simulink model "VCU_CS75_12_27_test"  (R2014a)
settings: Solver=FixedStepDiscrete  StartTime=0.0  StopTime=25  FixedStep=0.0005  RelTol=1e-3
undefined symbols (not defined in the file): D1, D2, D3, ecucoder_acal, ErrorSumMax1, ErrorSumMax2, ErrorSumMax3, I1, I2, I3, I_SW01_L, LaterlAngleCommand, LDW, P1, P2, P3, RemoteAcclPosition
libraries: simulink x913, ec5744lib x39
(part 3 of 30)

== system VCU_CS75_12_27_test/长安CS75底盘程序，20ms一次/Output/Subsystem/TransmitMessages11 ==
  GW_LCDAL_2EA : Subsystem
  GW_LCDAL_2EA_Ter : Terminator
  LCDAL_AudioWarningEnableStatus : Ground
  LCDAL_BSDLCAAlert : Ground
  LCDAL_BSDLCAEnableStatus : Ground
  LCDAL_BSDLCAStatus : Ground
  LCDAL_CTAAlert : Ground
  LCDAL_CTAEnableStatus : Ground
  LCDAL_CTAStatus : Ground
  LCDAL_LCATTCSettingStatus : Ground
  LCDAL_LockCtrlEnableStatus : Ground
  LCDAL_RCWAlert : Ground
  LCDAL_RCWEnableStatus : Ground
  LCDAL_RCWSoundEnableStatus : Ground
  LCDAL_RCWStatus : Ground
  LCDAL_SEAAlert : Ground
  LCDAL_SEAEnableStatus : Ground
  LCDAL_SEAStatus : Ground
  LCDAL_SystemStatus : Ground
  wires:
  GW_LCDAL_2EA/1(output) -> GW_LCDAL_2EA_Ter/1
  LCDAL_LCATTCSettingStatus/1 -> GW_LCDAL_2EA/17(LCDAL_LCATTCSettingStatus_in)
  LCDAL_LockCtrlEnableStatus/1 -> GW_LCDAL_2EA/16(LCDAL_LockCtrlEnableStatus_in)
  LCDAL_AudioWarningEnableStatus/1 -> GW_LCDAL_2EA/15(LCDAL_AudioWarningEnableStatus_in)
  LCDAL_SEAStatus/1 -> GW_LCDAL_2EA/14(LCDAL_SEAStatus_in)
  LCDAL_SEAAlert/1 -> GW_LCDAL_2EA/13(LCDAL_SEAAlert_in)
  LCDAL_SEAEnableStatus/1 -> GW_LCDAL_2EA/12(LCDAL_SEAEnableStatus_in)
  LCDAL_RCWSoundEnableStatus/1 -> GW_LCDAL_2EA/11(LCDAL_RCWSoundEnableStatus_in)
  LCDAL_RCWStatus/1 -> GW_LCDAL_2EA/10(LCDAL_RCWStatus_in)
  LCDAL_RCWAlert/1 -> GW_LCDAL_2EA/9(LCDAL_RCWAlert_in)
  LCDAL_RCWEnableStatus/1 -> GW_LCDAL_2EA/8(LCDAL_RCWEnableStatus_in)
  LCDAL_CTAStatus/1 -> GW_LCDAL_2EA/7(LCDAL_CTAStatus_in)
  LCDAL_CTAAlert/1 -> GW_LCDAL_2EA/6(LCDAL_CTAAlert_in)
  LCDAL_CTAEnableStatus/1 -> GW_LCDAL_2EA/5(LCDAL_CTAEnableStatus_in)
  LCDAL_BSDLCAStatus/1 -> GW_LCDAL_2EA/4(LCDAL_BSDLCAStatus_in)
  LCDAL_BSDLCAAlert/1 -> GW_LCDAL_2EA/3(LCDAL_BSDLCAAlert_in)
  LCDAL_BSDLCAEnableStatus/1 -> GW_LCDAL_2EA/2(LCDAL_BSDLCAEnableStatus_in)
  LCDAL_SystemStatus/1 -> GW_LCDAL_2EA/1(LCDAL_SystemStatus_in)

== system VCU_CS75_12_27_test/长安CS75底盘程序，20ms一次/Output/Subsystem/TransmitMessages13 ==
  GW_LCDAR_2FA : Subsystem
  GW_LCDAR_2FA_Ter : Terminator
  LCDAR_BSDLCAAlert : Ground
  LCDAR_BSDLCAStatus : Ground
  LCDAR_CTAAlert : Ground
  LCDAR_CTAStatus : Ground
  LCDAR_RCWAlert : Ground
  LCDAR_RCWStatus : Ground
  LCDAR_SEAAlert : Ground
  LCDAR_SEAStatus : Ground
  LCDAR_SystemStatus : Ground
  wires:
  LCDAR_SystemStatus/1 -> GW_LCDAR_2FA/1(LCDAR_SystemStatus_in)
  LCDAR_BSDLCAAlert/1 -> GW_LCDAR_2FA/2(LCDAR_BSDLCAAlert_in)
  LCDAR_BSDLCAStatus/1 -> GW_LCDAR_2FA/3(LCDAR_BSDLCAStatus_in)
  LCDAR_CTAAlert/1 -> GW_LCDAR_2FA/4(LCDAR_CTAAlert_in)
  LCDAR_CTAStatus/1 -> GW_LCDAR_2FA/5(LCDAR_CTAStatus_in)
  LCDAR_RCWAlert/1 -> GW_LCDAR_2FA/6(LCDAR_RCWAlert_in)
  LCDAR_RCWStatus/1 -> GW_LCDAR_2FA/7(LCDAR_RCWStatus_in)
  LCDAR_SEAAlert/1 -> GW_LCDAR_2FA/8(LCDAR_SEAAlert_in)
  LCDAR_SEAStatus/1 -> GW_LCDAR_2FA/9(LCDAR_SEAStatus_in)
  GW_LCDAR_2FA/1(output) -> GW_LCDAR_2FA_Ter/1

== system VCU_CS75_12_27_test/长安CS75底盘程序，20ms一次/Output/Subsystem/TransmitMessages14 ==
  CRC : Ground
  LAS_2AD : Subsystem
  LAS_2AD_Ter : Terminator
  LAS_DriverHandsOff : Ground
  LAS_IACCMode : Ground
  LAS_IACCTextInfoForDriver : Ground
  LAS_TargetBasedLateralCOntrol : Ground
  RollingConter : Ground
  wires:
  LAS_2AD/1(output) -> LAS_2AD_Ter/1
  CRC/1 -> LAS_2AD/6(CRC_in)
  RollingConter/1 -> LAS_2AD/5(RollingConter_in)
  LAS_IACCTextInfoForDriver/1 -> LAS_2AD/4(LAS_IACCTextInfoForDriver_in)
  LAS_IACCMode/1 -> LAS_2AD/3(LAS_IACCMode_in)
  LAS_DriverHandsOff/1 -> LAS_2AD/2(LAS_DriverHandsOff_in)
  LAS_TargetBasedLateralCOntrol/1 -> LAS_2AD/1(LAS_TargetBasedLateralCOntrol_in)

== system VCU_CS75_12_27_test/长安CS75底盘程序，20ms一次/Output/Subsystem/TransmitMessages2 ==
  ACC_3C5 : Subsystem
  ACC_3C5_Ter : Terminator
  ACC_TargetRange : Ground
  ACC_TargetType : Ground
  CRC : Ground
  RollingConter : Ground
  wires:
  ACC_TargetRange/1 -> ACC_3C5/1(ACC_TargetRange_in)
  ACC_TargetType/1 -> ACC_3C5/2(ACC_TargetType_in)
  RollingConter/1 -> ACC_3C5/3(RollingConter_in)
  CRC/1 -> ACC_3C5/4(CRC_in)
  ACC_3C5/1(output) -> ACC_3C5_Ter/1

== system VCU_CS75_12_27_test/长安CS75底盘程序，20ms一次/Output/Subsystem/TransmitMessages3 ==
  ACC_3D5 : Subsystem
  ACC_3D5_Ter : Terminator
  ACC_LeftTargetDection : Ground
  ACC_LeftTargetLatRange : Ground
  ACC_LeftTargetLngRange : Ground
  ACC_LeftTargetType : Ground
  ACC_RightTargetDection : Ground
  ACC_RightTargetLatRange : Ground
  ACC_RightTargetLngRange : Ground
  ACC_RightTargetType : Ground
  CRC : Ground
  RollingConter : Ground
  wires:
  ACC_LeftTargetLngRange/1 -> ACC_3D5/1(ACC_LeftTargetLngRange_in)
  ACC_RightTargetDection/1 -> ACC_3D5/2(ACC_RightTargetDection_in)
  ACC_LeftTargetDection/1 -> ACC_3D5/3(ACC_LeftTargetDection_in)
  ACC_LeftTargetType/1 -> ACC_3D5/4(ACC_LeftTargetType_in)
  ACC_LeftTargetLatRange/1 -> ACC_3D5/5(ACC_LeftTargetLatRange_in)
  ACC_RightTargetType/1 -> ACC_3D5/6(ACC_RightTargetType_in)
  ACC_RightTargetLatRange/1 -> ACC_3D5/7(ACC_RightTargetLatRange_in)
  ACC_RightTargetLngRange/1 -> ACC_3D5/8(ACC_RightTargetLngRange_in)
  RollingConter/1 -> ACC_3D5/9(RollingConter_in)
  CRC/1 -> ACC_3D5/10(CRC_in)
  ACC_3D5/1(output) -> ACC_3D5_Ter/1

== system VCU_CS75_12_27_test/长安CS75底盘程序，20ms一次/Output/Subsystem/TransmitMessages4 ==
  ACC_3E5 : Subsystem
  ACC_3E5_Ter : Terminator
  ACC_ACCObjEnableStatus : Ground
  ACC_AutoBrakeEnableStatus : Ground
  ACC_ControlType : Ground
  ACC_DistanceTarObj : Ground
  ACC_EPBReq : Ground
  ACC_FCWEnableStatus : Ground
  ACC_FCWSensityStatus : Ground
  ACC_ObjValid : Ground
  ACC_SetSpeedDisplay : Ground
  ACC_TimeGapSet : Ground
  ACC_takeoverRequesr : Ground
  CRC : Ground
  RollingConter : Ground
  wires:
  ACC_3E5/1(output) -> ACC_3E5_Ter/1
  CRC/1 -> ACC_3E5/13(CRC_in)
  ACC_AutoBrakeEnableStatus/1 -> ACC_3E5/12(ACC_AutoBrakeEnableStatus_in)
  ACC_EPBReq/1 -> ACC_3E5/11(ACC_EPBReq_in)
  RollingConter/1 -> ACC_3E5/10(RollingConter_in)
  ACC_FCWEnableStatus/1 -> ACC_3E5/9(ACC_FCWEnableStatus_in)
  ACC_FCWSensityStatus/1 -> ACC_3E5/8(ACC_FCWSensityStatus_in)
  ACC_ACCObjEnableStatus/1 -> ACC_3E5/7(ACC_ACCObjEnableStatus_in)
  ACC_takeoverRequesr/1 -> ACC_3E5/6(ACC_takeoverRequesr_in)
  ACC_ControlType/1 -> ACC_3E5/5(ACC_ControlType_in)
  ACC_DistanceTarObj/1 -> ACC_3E5/4(ACC_DistanceTarObj_in)
  ACC_TimeGapSet/1 -> ACC_3E5/3(ACC_TimeGapSet_in)
  ACC_ObjValid/1 -> ACC_3E5/2(ACC_ObjValid_in)
  ACC_SetSpeedDisplay/1 -> ACC_3E5/1(ACC_SetSpeedDisplay_in)

== system VCU_CS75_12_27_test/长安CS75底盘程序，20ms一次/Output/Subsystem/TransmitMessages5 ==
  ACC_3F5 : Subsystem
  ACC_3F5_Ter : Terminator
  ACC_AEBTargetLatRange : Ground
  ACC_AEBTargetLngRange : Ground
  ACC_AEBTargetRelSpeed : Ground
  ACC_HostPotentialTargetDetection : Ground
  ACC_HostPotentialTargetLatRng : Ground
  ACC_HostPotentialTargetLngRng : Ground
  ACC_HostPotentialTargetType : Ground
  CRC : Ground
  RollingConter : Ground
  wires:
  ACC_AEBTargetLngRange/1 -> ACC_3F5/1(ACC_AEBTargetLngRange_in)
  ACC_AEBTargetRelSpeed/1 -> ACC_3F5/2(ACC_AEBTargetRelSpeed_in)
  ACC_AEBTargetLatRange/1 -> ACC_3F5/3(ACC_AEBTargetLatRange_in)
  ACC_HostPotentialTargetLatRng/1 -> ACC_3F5/4(ACC_HostPotentialTargetLatRng_in)
  ACC_HostPotentialTargetDetection/1 -> ACC_3F5/5(ACC_HostPotentialTargetDetection_in)
  ACC_HostPotentialTargetLngRng/1 -> ACC_3F5/6(ACC_HostPotentialTargetLngRng_in)
  RollingConter/1 -> ACC_3F5/7(RollingConter_in)
  ACC_HostPotentialTargetType/1 -> ACC_3F5/8(ACC_HostPotentialTargetType_in)
  CRC/1 -> ACC_3F5/9(CRC_in)
  ACC_3F5/1(output) -> ACC_3F5_Ter/1

== system VCU_CS75_12_27_test/长安CS75底盘程序，20ms一次/Output/Subsystem/TransmitMessages7 ==
  APA_29A : Subsystem
  APA_29A_Ter : Terminator
  APA_ActivationStatus : Ground
  APA_Checksum : Ground
  APA_EPBrequest : Ground
  APA_EPBrequestValid : Ground
  APA_GearReqValid : Ground
  APA_LSCAction : Ground
  APA_RollingCounter : Ground
  APA_TargetAcceleration : Ground
  APA_TargetAccelerationValid : Ground
  APA_TranShiftReqValid : Ground
  APA_TranShiftRequest : Ground
  wires:
  APA_EPBrequest/1 -> APA_29A/1(APA_EPBrequest_in)
  APA_EPBrequestValid/1 -> APA_29A/2(APA_EPBrequestValid_in)
  APA_TranShiftReqValid/1 -> APA_29A/3(APA_TranShiftReqValid_in)
  APA_TranShiftRequest/1 -> APA_29A/4(APA_TranShiftRequest_in)
  APA_TargetAcceleration/1 -> APA_29A/5(APA_TargetAcceleration_in)
  APA_TargetAccelerationValid/1 -> APA_29A/6(APA_TargetAccelerationValid_in)
  APA_GearReqValid/1 -> APA_29A/7(APA_GearReqValid_in)
  APA_LSCAction/1 -> APA_29A/8(APA_LSCAction_in)
  APA_ActivationStatus/1 -> APA_29A/9(APA_ActivationStatus_in)
  APA_RollingCounter/1 -> APA_29A/10(APA_RollingCounter_in)
  APA_Checksum/1 -> APA_29A/11(APA_Checksum_in)
  APA_29A/1(output) -> APA_29A_Ter/1

== system VCU_CS75_12_27_test/长安CS75底盘程序，20ms一次/Output/Subsystem/TransmitMessages8 ==
  APA_2D4 : Subsystem
  APA_2D4_Ter : Terminator
  APA_APAStatus : Ground
  APA_ReleasePressureReq : Ground
  CRC : Ground
  RollingConter : Ground
  wires:
  APA_APAStatus/1 -> APA_2D4/1(APA_APAStatus_in)
  APA_ReleasePressureReq/1 -> APA_2D4/2(APA_ReleasePressureReq_in)
  RollingConter/1 -> APA_2D4/3(RollingConter_in)
  CRC/1 -> APA_2D4/4(CRC_in)
  APA_2D4/1(output) -> APA_2D4_Ter/1

== system VCU_CS75_12_27_test/长安CS75底盘程序，20ms一次/Input/CAN0_Rx/a1_211/ReceiveMessages ==
  In1 : Inport
  In2 : Inport  Port=2
  function : TriggerPort  TriggerType=function-call
  Subsystem : Subsystem
  A1_211 : Outport
  wires:
  In1/1 -> Subsystem/Enable
  In2/1 -> Subsystem/1(input)
  Subsystem/1(A1_211) -> A1_211/1

== system VCU_CS75_12_27_test/长安CS75底盘程序，20ms一次/Input/CAN1_Rx/BCM_288/ReceiveMessages ==
  In1 : Inport
  In2 : Inport  Port=2
  function : TriggerPort  TriggerType=function-call
  Subsystem : Subsystem
  BCM_288 : Outport
  wires:
  Subsystem/1(BCM_288) -> BCM_288/1
  In2/1 -> Subsystem/1(input)
  In1/1 -> Subsystem/Enable

== system VCU_CS75_12_27_test/长安CS75底盘程序，20ms一次/Input/CAN1_Rx/BCM_328/ReceiveMessages ==
  In1 : Inport
  In2 : Inport  Port=2
  function : TriggerPort  TriggerType=function-call
  Subsystem : Subsystem
  BCM_328 : Outport
  wires:
  In1/1 -> Subsystem/Enable
  In2/1 -> Subsystem/1(input)
  Subsystem/1(BCM_328) -> BCM_328/1

== system VCU_CS75_12_27_test/长安CS75底盘程序，20ms一次/Input/CAN1_Rx/BCM_348/ReceiveMessages ==
  In1 : Inport
  In2 : Inport  Port=2
  function : TriggerPort  TriggerType=function-call
  Subsystem : Subsystem
  BCM_348 : Outport
  wires:
  Subsystem/1(BCM_348) -> BCM_348/1
  In2/1 -> Subsystem/1(input)
  In1/1 -> Subsystem/Enable

== system VCU_CS75_12_27_test/长安CS75底盘程序，20ms一次/Input/CAN1_Rx/BCM_3DF/ReceiveMessages ==
  In1 : Inport
  In2 : Inport  Port=2
  function : TriggerPort  TriggerType=function-call
  Subsystem : Subsystem
  BCM_3DF : Outport
  wires:
  In1/1 -> Subsystem/Enable
  In2/1 -> Subsystem/1(input)
  Subsystem/1(BCM_3DF) -> BCM_3DF/1

== system VCU_CS75_12_27_test/长安CS75底盘程序，20ms一次/Input/CAN1_Rx/EMS_205/ReceiveMessages ==
  In1 : Inport
  In2 : Inport  Port=2
  function : TriggerPort  TriggerType=function-call
  Subsystem : Subsystem
  EMS_205 : Outport
  wires:
  In1/1 -> Subsystem/Enable
  In2/1 -> Subsystem/1(input)
  Subsystem/1(EMS_205) -> EMS_205/1

== system VCU_CS75_12_27_test/长安CS75底盘程序，20ms一次/Input/CAN1_Rx/EMS_255/ReceiveMessages ==
  In1 : Inport
  In2 : Inport  Port=2
  function : TriggerPort  TriggerType=function-call
  Subsystem : Subsystem
  EMS_255 : Outport
  wires:
  Subsystem/1(EMS_255) -> EMS_255/1
  In2/1 -> Subsystem/1(input)
  In1/1 -> Subsystem/Enable

== system VCU_CS75_12_27_test/长安CS75底盘程序，20ms一次/Input/CAN1_Rx/EMS_265/ReceiveMessages ==
  In1 : Inport
  In2 : Inport  Port=2
  function : TriggerPort  TriggerType=function-call
  Subsystem : Subsystem
  EMS_265 : Outport
  wires:
  In1/1 -> Subsystem/Enable
  In2/1 -> Subsystem/1(input)
  Subsystem/1(EMS_265) -> EMS_265/1

== system VCU_CS75_12_27_test/长安CS75底盘程序，20ms一次/Input/CAN1_Rx/EMS_276/ReceiveMessages ==
  In1 : Inport
  In2 : Inport  Port=2
  function : TriggerPort  TriggerType=function-call
  Subsystem : Subsystem
  EMS_276 : Outport
  wires:
  Subsystem/1(EMS_276) -> EMS_276/1
  In2/1 -> Subsystem/1(input)
  In1/1 -> Subsystem/Enable

== system VCU_CS75_12_27_test/长安CS75底盘程序，20ms一次/Input/CAN1_Rx/EPB_256/ReceiveMessages ==
  In1 : Inport
  In2 : Inport  Port=2
  function : TriggerPort  TriggerType=function-call
  Subsystem : Subsystem
  EMS_256 : Outport
  wires:
  In1/1 -> Subsystem/Enable
  In2/1 -> Subsystem/1(input)
  Subsystem/1(EPB_256) -> EMS_256/1

== system VCU_CS75_12_27_test/长安CS75底盘程序，20ms一次/Input/CAN1_Rx/EPS_20A/ReceiveMessages ==
  In1 : Inport
  In2 : Inport  Port=2
  function : TriggerPort  TriggerType=function-call
  Subsystem : Subsystem
  EPS_20A : Outport
  wires:
  Subsystem/1(EPS_20A) -> EPS_20A/1
  In2/1 -> Subsystem/1(input)
  In1/1 -> Subsystem/Enable

== system VCU_CS75_12_27_test/长安CS75底盘程序，20ms一次/Input/CAN1_Rx/EPS_21A/ReceiveMessages ==
  In1 : Inport
  In2 : Inport  Port=2
  function : TriggerPort  TriggerType=function-call
  Subsystem : Subsystem
  EPS_21A : Outport
  wires:
  In1/1 -> Subsystem/Enable
  In2/1 -> Subsystem/1(input)
  Subsystem/1(EPS_21A) -> EPS_21A/1

== system VCU_CS75_12_27_test/长安CS75底盘程序，20ms一次/Input/CAN1_Rx/ESP_277/ReceiveMessages ==
  In1 : Inport
  In2 : Inport  Port=2
  function : TriggerPort  TriggerType=function-call
  Subsystem : Subsystem
  ESP_277 : Outport
  wires:
  Subsystem/1(ESP_277) -> ESP_277/1
  In2/1 -> Subsystem/1(input)
  In1/1 -> Subsystem/Enable

== system VCU_CS75_12_27_test/长安CS75底盘程序，20ms一次/Input/CAN1_Rx/ESP_280/ReceiveMessages ==
  In1 : Inport
  In2 : Inport  Port=2
  function : TriggerPort  TriggerType=function-call
  Subsystem : Subsystem
  ESP_280 : Outport
  wires:
  In1/1 -> Subsystem/Enable
  In2/1 -> Subsystem/1(input)
  Subsystem/1(ESP_280) -> ESP_280/1

== system VCU_CS75_12_27_test/长安CS75底盘程序，20ms一次/Input/CAN1_Rx/ESP_281/ReceiveMessages ==
  In1 : Inport
  In2 : Inport  Port=2
  function : TriggerPort  TriggerType=function-call
  Subsystem : Subsystem
  ESP_281 : Outport
  wires:
  Subsystem/1(ESP_281) -> ESP_281/1
  In2/1 -> Subsystem/1(input)
  In1/1 -> Subsystem/Enable

== system VCU_CS75_12_27_test/长安CS75底盘程序，20ms一次/Input/CAN1_Rx/ESP_287/ReceiveMessages ==
  In1 : Inport
  In2 : Inport  Port=2
  function : TriggerPort  TriggerType=function-call
  Subsystem : Subsystem
  ESP_287 : Outport
  wires:
  In1/1 -> Subsystem/Enable
  In2/1 -> Subsystem/1(input)
  Subsystem/1(ESP_287) -> ESP_287/1

== system VCU_CS75_12_27_test/长安CS75底盘程序，20ms一次/Input/CAN1_Rx/GW_20B/ReceiveMessages ==
  In1 : Inport
  In2 : Inport  Port=2
  function : TriggerPort  TriggerType=function-call
  Subsystem : Subsystem
  GW_20B : Outport
  wires:
  Subsystem/1(GW_20B) -> GW_20B/1
  In2/1 -> Subsystem/1(input)
  In1/1 -> Subsystem/Enable

== system VCU_CS75_12_27_test/长安CS75底盘程序，20ms一次/Input/CAN1_Rx/GW_308/ReceiveMessages ==
  In1 : Inport
  In2 : Inport  Port=2
  function : TriggerPort  TriggerType=function-call
  Subsystem : Subsystem
  GW_308 : Outport
  wires:
  Subsystem/1(GW_308) -> GW_308/1
  In2/1 -> Subsystem/1(input)
  In1/1 -> Subsystem/Enable

== system VCU_CS75_12_27_test/长安CS75底盘程序，20ms一次/Input/CAN1_Rx/GW_332/ReceiveMessages ==
  In1 : Inport
  In2 : Inport  Port=2
  function : TriggerPort  TriggerType=function-call
  Subsystem : Subsystem
  GW_332 : Outport
  wires:
  In1/1 -> Subsystem/Enable
  In2/1 -> Subsystem/1(input)
  Subsystem/1(GW_332) -> GW_332/1

== system VCU_CS75_12_27_test/长安CS75底盘程序，20ms一次/Input/CAN1_Rx/GW_376/ReceiveMessages ==
  In1 : Inport
  In2 : Inport  Port=2
  function : TriggerPort  TriggerType=function-call
  Subsystem : Subsystem
  GW_376 : Outport
  wires:
  In1/1 -> Subsystem/Enable
  In2/1 -> Subsystem/1(input)
  Subsystem/1(GW_376) -> GW_376/1

== system VCU_CS75_12_27_test/长安CS75底盘程序，20ms一次/Input/CAN1_Rx/GW_3A2/ReceiveMessages ==
  In1 : Inport
  In2 : Inport  Port=2
  function : TriggerPort  TriggerType=function-call
  Subsystem : Subsystem
  GW_3A2 : Outport
  wires:
  Subsystem/1(GW_3A2) -> GW_3A2/1
  In2/1 -> Subsystem/1(input)
  In1/1 -> Subsystem/Enable

== system VCU_CS75_12_27_test/长安CS75底盘程序，20ms一次/Input/CAN1_Rx/GW_567/ReceiveMessages ==
  In1 : Inport
  In2 : Inport  Port=2
  function : TriggerPort  TriggerType=function-call
  Subsystem : Subsystem
  GW_567 : Outport
  wires:
  In1/1 -> Subsystem/Enable
  In2/1 -> Subsystem/1(input)
  Subsystem/1(GW_567) -> GW_567/1

== system VCU_CS75_12_27_test/长安CS75底盘程序，20ms一次/Input/CAN1_Rx/HU_GPS_500/ReceiveMessages ==
  In1 : Inport
  In2 : Inport  Port=2
  function : TriggerPort  TriggerType=function-call
  Subsystem : Subsystem
  HU_GPS_500 : Outport
  wires:
  Subsystem/1(HU_GPS_500) -> HU_GPS_500/1
  In2/1 -> Subsystem/1(input)
  In1/1 -> Subsystem/Enable

== system VCU_CS75_12_27_test/长安CS75底盘程序，20ms一次/Input/CAN1_Rx/LAS_36E/ReceiveMessages ==
  In1 : Inport
  In2 : Inport  Port=2
  function : TriggerPort  TriggerType=function-call
  Subsystem : Subsystem
  LAS_36E : Outport
  wires:
  In1/1 -> Subsystem/Enable
  In2/1 -> Subsystem/1(input)
  Subsystem/1(LAS_36E) -> LAS_36E/1

== system VCU_CS75_12_27_test/长安CS75底盘程序，20ms一次/Input/CAN1_Rx/SAS_108/ReceiveMessages ==
  In1 : Inport
  In2 : Inport  Port=2
  function : TriggerPort  TriggerType=function-call
  Subsystem : Subsystem
  SAS_108 : Outport
  wires:
  Subsystem/1(SAS_108) -> SAS_108/1
  In2/1 -> Subsystem/1(input)
  In1/1 -> Subsystem/Enable

== system VCU_CS75_12_27_test/长安CS75底盘程序，20ms一次/Input/CAN1_Rx/SCM_3B8/ReceiveMessages ==
  In1 : Inport
  In2 : Inport  Port=2
  function : TriggerPort  TriggerType=function-call
  Subsystem : Subsystem
  SCM_3B8 : Outport
  wires:
  In1/1 -> Subsystem/Enable
  In2/1 -> Subsystem/1(input)
  Subsystem/1(SCM_3B8) -> SCM_3B8/1

== system VCU_CS75_12_27_test/长安CS75底盘程序，20ms一次/Input/CAN1_Rx/SRS_005/ReceiveMessages ==
  In1 : Inport
  In2 : Inport  Port=2
  function : TriggerPort  TriggerType=function-call
  Subsystem : Subsystem
  SRS_005 : Outport
  wires:
  Subsystem/1(SRS_005) -> SRS_005/1
  In2/1 -> Subsystem/1(input)
  In1/1 -> Subsystem/Enable

== system VCU_CS75_12_27_test/长安CS75底盘程序，20ms一次/Input/CAN1_Rx/TCU_286/ReceiveMessages ==
  In1 : Inport
  In2 : Inport  Port=2
  function : TriggerPort  TriggerType=function-call
  Subsystem : Subsystem
  TCU_286 : Outport
  wires:
  In1/1 -> Subsystem/Enable
  In2/1 -> Subsystem/1(input)
  Subsystem/1(TCU_286) -> TCU_286/1

== system VCU_CS75_12_27_test/长安CS75底盘程序，20ms一次/Input/DBC转化的messages（存底）/ReceiveMessages/EMS_205 ==
  input : Inport
  Demux : Demux  Outputs=8
  EMS_CheckSum_205_Ad : Sum
  EMS_CheckSum_205_Convert : DataTypeConversion  OutDataTypeStr=uint32
  EMS_CheckSum_205_F : Gain
  EMS_CheckSum_205_L : simulink/Logic and Bit Operations/Bitwise Operator  logicop=AND  UseBitMask=on  BitMask=240  BitMaskRealWorld=Stored Integer
  EMS_CheckSum_205_O : Constant  Value=0  OutDataTypeStr=single
  EMS_CheckSum_205_S : ArithShift  BitShiftNumber=4
  EMS_CheckSum_205_Sub : Subsystem
  EMS_CheckSum_205_sat : Saturate  UpperLimit=15  LowerLimit=0
  EMS_CheckSum_205cv : DataTypeConversion
  EMS_ESPTorqReuestAvailability_Ad : Sum
  EMS_ESPTorqReuestAvailability_Convert : DataTypeConversion  OutDataTypeStr=uint32
  EMS_ESPTorqReuestAvailability_F : Gain
  EMS_ESPTorqReuestAvailability_L : simulink/Logic and Bit Operations/Bitwise Operator  logicop=AND  UseBitMask=on  BitMask=2  BitMaskRealWorld=Stored Integer
  EMS_ESPTorqReuestAvailability_O : Constant  Value=0  OutDataTypeStr=single
  EMS_ESPTorqReuestAvailability_S : ArithShift  BitShiftNumber=1
  EMS_ESPTorqReuestAvailability_Sub : Subsystem
  EMS_ESPTorqReuestAvailability_sat : Saturate  UpperLimit=1  LowerLimit=0
  EMS_ESPTorqReuestAvailabilitycv : DataTypeConversion
  EMS_FrictionalTorq_Ad : Sum
  EMS_FrictionalTorq_Convert : DataTypeConversion  OutDataTypeStr=uint32
  EMS_FrictionalTorq_F : Gain  Gain=0.001526
  EMS_FrictionalTorq_L : simulink/Logic and Bit Operations/Bitwise Operator  logicop=AND  UseBitMask=on  BitMask=65535  BitMaskRealWorld=Stored Integer
  EMS_FrictionalTorq_O : Constant  Value=0  OutDataTypeStr=single
  EMS_FrictionalTorq_S : ArithShift
  EMS_FrictionalTorq_Sub : Subsystem
  EMS_FrictionalTorq_sat : Saturate  UpperLimit=99.9988  LowerLimit=0
  EMS_FrictionalTorqcv : DataTypeConversion
  EMS_FrictionalTorqinput4_Ad : Sum
  EMS_FrictionalTorqinput4_C : Constant  Value=256
  EMS_FrictionalTorqinput4_P : Product
  EMS_IndicatedDriverReqTorq_Ad : Sum
  EMS_IndicatedDriverReqTorq_Convert : DataTypeConversion  OutDataTypeStr=uint32
  EMS_IndicatedDriverReqTorq_F : Gain  Gain=0.001526
  EMS_IndicatedDriverReqTorq_L : simulink/Logic and Bit Operations/Bitwise Operator  logicop=AND  UseBitMask=on  BitMask=65535  BitMaskRealWorld=Stored Integer
  EMS_IndicatedDriverReqTorq_O : Constant  Value=0  OutDataTypeStr=single
  EMS_IndicatedDriverReqTorq_S : ArithShift
  EMS_IndicatedDriverReqTorq_Sub : Subsystem
  EMS_IndicatedDriverReqTorq_sat : Saturate  UpperLimit=99.9988  LowerLimit=0
  EMS_IndicatedDriverReqTorqcv : DataTypeConversion
  EMS_IndicatedDriverReqTorqinput2_Ad : Sum
  EMS_IndicatedDriverReqTorqinput2_C : Constant  Value=256
  EMS_IndicatedDriverReqTorqinput2_P : Product
  EMS_IndicatedRealEngTorq_Ad : Sum
  EMS_IndicatedRealEngTorq_Convert : DataTypeConversion  OutDataTypeStr=uint32
  EMS_IndicatedRealEngTorq_F : Gain  Gain=0.001526
  EMS_IndicatedRealEngTorq_L : simulink/Logic and Bit Operations/Bitwise Operator  logicop=AND  UseBitMask=on  BitMask=65535  BitMaskRealWorld=Stored Integer
  EMS_IndicatedRealEngTorq_O : Constant  Value=0  OutDataTypeStr=single
  EMS_IndicatedRealEngTorq_S : ArithShift
  EMS_IndicatedRealEngTorq_Sub : Subsystem
  EMS_IndicatedRealEngTorq_sat : Saturate  UpperLimit=99.9988  LowerLimit=0
  EMS_IndicatedRealEngTorqcv : DataTypeConversion
  EMS_IndicatedRealEngTorqinput6_Ad : Sum
  EMS_IndicatedRealEngTorqinput6_C : Constant  Value=256
  EMS_IndicatedRealEngTorqinput6_P : Product
  EMS_RollingCounter_id205_Ad : Sum
  EMS_RollingCounter_id205_Convert : DataTypeConversion  OutDataTypeStr=uint32
  EMS_RollingCounter_id205_F : Gain
  EMS_RollingCounter_id205_L : simulink/Logic and Bit Operations/Bitwise Operator  logicop=AND  UseBitMask=on  BitMask=15  BitMaskRealWorld=Stored Integer
  EMS_RollingCounter_id205_O : Constant  Value=0  OutDataTypeStr=single
  EMS_RollingCounter_id205_S : ArithShift
  EMS_RollingCounter_id205_Sub : Subsystem
  EMS_RollingCounter_id205_sat : Saturate  UpperLimit=15  LowerLimit=0
  EMS_RollingCounter_id205cv : DataTypeConversion
  EMS_TorqFailure_Ad : Sum
  EMS_TorqFailure_Convert : DataTypeConversion  OutDataTypeStr=uint32
  EMS_TorqFailure_F : Gain
  EMS_TorqFailure_L : simulink/Logic and Bit Operations/Bitwise Operator  logicop=AND  UseBitMask=on  BitMask=128  BitMaskRealWorld=Stored Integer
  EMS_TorqFailure_O : Constant  Value=0  OutDataTypeStr=single
  EMS_TorqFailure_S : ArithShift  BitShiftNumber=7
  EMS_TorqFailure_Sub : Subsystem
  EMS_TorqFailure_sat : Saturate  UpperLimit=1  LowerLimit=0
  EMS_TorqFailurecv : DataTypeConversion
  EMS_ESPTorqReuestAvailability_Out : Outport
  EMS_TorqFailure_Out : Outport  Port=2
  EMS_IndicatedDriverReqTorq_Out : Outport  Port=3
  EMS_FrictionalTorq_Out : Outport  Port=4
  EMS_IndicatedRealEngTorq_Out : Outport  Port=5
  EMS_RollingCounter_id205_Out : Outport  Port=6
  EMS_CheckSum_205_Out : Outport  Port=7
  wires:
  EMS_ESPTorqReuestAvailability_F/1 -> EMS_ESPTorqReuestAvailability_Ad/1
  EMS_ESPTorqReuestAvailability_O/1 -> EMS_ESPTorqReuestAvailability_Ad/2
  EMS_ESPTorqReuestAvailability_Ad/1 -> EMS_ESPTorqReuestAvailability_sat/1
  EMS_ESPTorqReuestAvailability_sat/1 -> EMS_ESPTorqReuestAvailability_Out/1
  Demux/1 -> EMS_ESPTorqReuestAvailability_Sub/1(In1), EMS_TorqFailure_Sub/1(In1)
  EMS_ESPTorqReuestAvailability_Sub/1(Out1) -> EMS_ESPTorqReuestAvailability_Convert/1
  EMS_ESPTorqReuestAvailability_Convert/1 -> EMS_ESPTorqReuestAvailability_L/1
  EMS_ESPTorqReuestAvailability_L/1 -> EMS_ESPTorqReuestAvailability_S/1
  EMS_ESPTorqReuestAvailability_S/1 -> EMS_ESPTorqReuestAvailabilitycv/1
  EMS_ESPTorqReuestAvailabilitycv/1 -> EMS_ESPTorqReuestAvailability_F/1
  EMS_TorqFailure_F/1 -> EMS_TorqFailure_Ad/1
  EMS_TorqFailure_O/1 -> EMS_TorqFailure_Ad/2
  EMS_TorqFailure_Ad/1 -> EMS_TorqFailure_sat/1
  EMS_TorqFailure_sat/1 -> EMS_TorqFailure_Out/1
  EMS_TorqFailure_Sub/1(Out1) -> EMS_TorqFailure_Convert/1
  EMS_TorqFailure_Convert/1 -> EMS_TorqFailure_L/1
  EMS_TorqFailure_L/1 -> EMS_TorqFailure_S/1
  EMS_TorqFailure_S/1 -> EMS_TorqFailurecv/1
  EMS_TorqFailurecv/1 -> EMS_TorqFailure_F/1
  EMS_IndicatedDriverReqTorq_F/1 -> EMS_IndicatedDriverReqTorq_Ad/1
  EMS_IndicatedDriverReqTorq_O/1 -> EMS_IndicatedDriverReqTorq_Ad/2
  EMS_IndicatedDriverReqTorq_Ad/1 -> EMS_IndicatedDriverReqTorq_sat/1
  EMS_IndicatedDriverReqTorq_sat/1 -> EMS_IndicatedDriverReqTorq_Out/1
  Demux/2 -> EMS_IndicatedDriverReqTorqinput2_P/1
  EMS_IndicatedDriverReqTorqinput2_C/1 -> EMS_IndicatedDriverReqTorqinput2_P/2
  EMS_IndicatedDriverReqTorqinput2_P/1 -> EMS_IndicatedDriverReqTorqinput2_Ad/1
  Demux/3 -> EMS_IndicatedDriverReqTorqinput2_Ad/2
  EMS_IndicatedDriverReqTorqinput2_Ad/1 -> EMS_IndicatedDriverReqTorq_Sub/1(In1)
  EMS_IndicatedDriverReqTorq_Sub/1(Out1) -> EMS_IndicatedDriverReqTorq_Convert/1
  EMS_IndicatedDriverReqTorq_Convert/1 -> EMS_IndicatedDriverReqTorq_L/1
  EMS_IndicatedDriverReqTorq_L/1 -> EMS_IndicatedDriverReqTorq_S/1
  EMS_IndicatedDriverReqTorq_S/1 -> EMS_IndicatedDriverReqTorqcv/1
  EMS_IndicatedDriverReqTorqcv/1 -> EMS_IndicatedDriverReqTorq_F/1
  EMS_FrictionalTorq_F/1 -> EMS_FrictionalTorq_Ad/1
  EMS_FrictionalTorq_O/1 -> EMS_FrictionalTorq_Ad/2
  EMS_FrictionalTorq_Ad/1 -> EMS_FrictionalTorq_sat/1
  EMS_FrictionalTorq_sat/1 -> EMS_FrictionalTorq_Out/1
  Demux/4 -> EMS_FrictionalTorqinput4_P/1
  EMS_FrictionalTorqinput4_C/1 -> EMS_FrictionalTorqinput4_P/2
  EMS_FrictionalTorqinput4_P/1 -> EMS_FrictionalTorqinput4_Ad/1
  Demux/5 -> EMS_FrictionalTorqinput4_Ad/2
  EMS_FrictionalTorqinput4_Ad/1 -> EMS_FrictionalTorq_Sub/1(In1)
  EMS_FrictionalTorq_Sub/1(Out1) -> EMS_FrictionalTorq_Convert/1
  EMS_FrictionalTorq_Convert/1 -> EMS_FrictionalTorq_L/1
  EMS_FrictionalTorq_L/1 -> EMS_FrictionalTorq_S/1
  EMS_FrictionalTorq_S/1 -> EMS_FrictionalTorqcv/1
  EMS_FrictionalTorqcv/1 -> EMS_FrictionalTorq_F/1
  EMS_IndicatedRealEngTorq_F/1 -> EMS_IndicatedRealEngTorq_Ad/1
  EMS_IndicatedRealEngTorq_O/1 -> EMS_IndicatedRealEngTorq_Ad/2
  EMS_IndicatedRealEngTorq_Ad/1 -> EMS_IndicatedRealEngTorq_sat/1
  EMS_IndicatedRealEngTorq_sat/1 -> EMS_IndicatedRealEngTorq_Out/1
  Demux/6 -> EMS_IndicatedRealEngTorqinput6_P/1
  EMS_IndicatedRealEngTorqinput6_C/1 -> EMS_IndicatedRealEngTorqinput6_P/2
  EMS_IndicatedRealEngTorqinput6_P/1 -> EMS_IndicatedRealEngTorqinput6_Ad/1
  Demux/7 -> EMS_IndicatedRealEngTorqinput6_Ad/2
  EMS_IndicatedRealEngTorqinput6_Ad/1 -> EMS_IndicatedRealEngTorq_Sub/1(In1)
  EMS_IndicatedRealEngTorq_Sub/1(Out1) -> EMS_IndicatedRealEngTorq_Convert/1
  EMS_IndicatedRealEngTorq_Convert/1 -> EMS_IndicatedRealEngTorq_L/1
  EMS_IndicatedRealEngTorq_L/1 -> EMS_IndicatedRealEngTorq_S/1
  EMS_IndicatedRealEngTorq_S/1 -> EMS_IndicatedRealEngTorqcv/1
  EMS_IndicatedRealEngTorqcv/1 -> EMS_IndicatedRealEngTorq_F/1
  EMS_RollingCounter_id205_F/1 -> EMS_RollingCounter_id205_Ad/1
  EMS_RollingCounter_id205_O/1 -> EMS_RollingCounter_id205_Ad/2
  EMS_RollingCounter_id205_Ad/1 -> EMS_RollingCounter_id205_sat/1
  EMS_RollingCounter_id205_sat/1 -> EMS_RollingCounter_id205_Out/1
  Demux/8 -> EMS_RollingCounter_id205_Sub/1(In1), EMS_CheckSum_205_Sub/1(In1)
  EMS_RollingCounter_id205_Sub/1(Out1) -> EMS_RollingCounter_id205_Convert/1
  EMS_RollingCounter_id205_Convert/1 -> EMS_RollingCounter_id205_L/1
  EMS_RollingCounter_id205_L/1 -> EMS_RollingCounter_id205_S/1
  EMS_RollingCounter_id205_S/1 -> EMS_RollingCounter_id205cv/1
  EMS_RollingCounter_id205cv/1 -> EMS_RollingCounter_id205_F/1
  EMS_CheckSum_205_F/1 -> EMS_CheckSum_205_Ad/1
  EMS_CheckSum_205_O/1 -> EMS_CheckSum_205_Ad/2
  EMS_CheckSum_205_Ad/1 -> EMS_CheckSum_205_sat/1
  EMS_CheckSum_205_sat/1 -> EMS_CheckSum_205_Out/1
  EMS_CheckSum_205_Sub/1(Out1) -> EMS_CheckSum_205_Convert/1
  EMS_CheckSum_205_Convert/1 -> EMS_CheckSum_205_L/1
  EMS_CheckSum_205_L/1 -> EMS_CheckSum_205_S/1
  EMS_CheckSum_205_S/1 -> EMS_CheckSum_205cv/1
  EMS_CheckSum_205cv/1 -> EMS_CheckSum_205_F/1
  input/1 -> Demux/1

== system VCU_CS75_12_27_test/长安CS75底盘程序，20ms一次/Input/DBC转化的messages（存底）/ReceiveMessages1/EMS_255 ==
  input : Inport
  Demux : Demux  Outputs=8
  EMS_AccPedal_Ad : Sum
  EMS_AccPedal_Convert : DataTypeConversion  OutDataTypeStr=uint32
  EMS_AccPedal_F : Gain  Gain=0.392
  EMS_AccPedal_L : simulink/Logic and Bit Operations/Bitwise Operator  logicop=AND  UseBitMask=on  BitMask=255  BitMaskRealWorld=Stored Integer
  EMS_AccPedal_O : Constant  Value=0  OutDataTypeStr=single
  EMS_AccPedal_S : ArithShift
  EMS_AccPedal_Sub : Subsystem
  EMS_AccPedal_sat : Saturate  UpperLimit=99.568  LowerLimit=0
  EMS_AccPedalcv : DataTypeConversion
  EMS_AccpedelError_Ad : Sum
  EMS_AccpedelError_Convert : DataTypeConversion  OutDataTypeStr=uint32
  EMS_AccpedelError_F : Gain
  EMS_AccpedelError_L : simulink/Logic and Bit Operations/Bitwise Operator  logicop=AND  UseBitMask=on  BitMask=4  BitMaskRealWorld=Stored Integer
  EMS_AccpedelError_O : Constant  Value=0  OutDataTypeStr=single
  EMS_AccpedelError_S : ArithShift  BitShiftNumber=2
  EMS_AccpedelError_Sub : Subsystem
  EMS_AccpedelError_sat : Saturate  UpperLimit=1  LowerLimit=0
  EMS_AccpedelErrorcv : DataTypeConversion
  EMS_BrakePedalStatus_Ad : Sum
  EMS_BrakePedalStatus_Convert : DataTypeConversion  OutDataTypeStr=uint32
  EMS_BrakePedalStatus_F : Gain
  EMS_BrakePedalStatus_L : simulink/Logic and Bit Operations/Bitwise Operator  logicop=AND  UseBitMask=on  BitMask=192  BitMaskRealWorld=Stored Integer
  EMS_BrakePedalStatus_O : Constant  Value=0  OutDataTypeStr=single
  EMS_BrakePedalStatus_S : ArithShift  BitShiftNumber=6
  EMS_BrakePedalStatus_Sub : Subsystem
  EMS_BrakePedalStatus_sat : Saturate  UpperLimit=3  LowerLimit=0
  EMS_BrakePedalStatuscv : DataTypeConversion
  EMS_CheckSum_255_Ad : Sum
  EMS_CheckSum_255_Convert : DataTypeConversion  OutDataTypeStr=uint32
  EMS_CheckSum_255_F : Gain
  EMS_CheckSum_255_L : simulink/Logic and Bit Operations/Bitwise Operator  logicop=AND  UseBitMask=on  BitMask=240  BitMaskRealWorld=Stored Integer
  EMS_CheckSum_255_O : Constant  Value=0  OutDataTypeStr=single
  EMS_CheckSum_255_S : ArithShift  BitShiftNumber=4
  EMS_CheckSum_255_Sub : Subsystem
  EMS_CheckSum_255_sat : Saturate  UpperLimit=15  LowerLimit=0
  EMS_CheckSum_255cv : DataTypeConversion
  EMS_EngineSpeedError_Ad : Sum
  EMS_EngineSpeedError_Convert : DataTypeConversion  OutDataTypeStr=uint32
  EMS_EngineSpeedError_F : Gain
  EMS_EngineSpeedError_L : simulink/Logic and Bit Operations/Bitwise Operator  logicop=AND  UseBitMask=on  BitMask=16  BitMaskRealWorld=Stored Integer
  EMS_EngineSpeedError_O : Constant  Value=0  OutDataTypeStr=single
  EMS_EngineSpeedError_S : ArithShift  BitShiftNumber=4
  EMS_EngineSpeedError_Sub : Subsystem
  EMS_EngineSpeedError_sat : Saturate  UpperLimit=1  LowerLimit=0
  EMS_EngineSpeedErrorcv : DataTypeConversion
  EMS_EngineSpeed_Ad : Sum
  EMS_EngineSpeed_Convert : DataTypeConversion  OutDataTypeStr=uint32
  EMS_EngineSpeed_F : Gain  Gain=0.25
  EMS_EngineSpeed_L : simulink/Logic and Bit Operations/Bitwise Operator  logicop=AND  UseBitMask=on  BitMask=65535  BitMaskRealWorld=Stored Integer
  EMS_EngineSpeed_O : Constant  Value=0  OutDataTypeStr=single
  EMS_EngineSpeed_S : ArithShift
  EMS_EngineSpeed_Sub : Subsystem
  EMS_EngineSpeed_sat : Saturate  UpperLimit=16383.5  LowerLimit=0
  EMS_EngineSpeedcv : DataTypeConversion
  EMS_EngineSpeedinput3_Ad : Sum
  EMS_EngineSpeedinput3_C : Constant  Value=256
  EMS_EngineSpeedinput3_P : Product
  EMS_RollingCounter_id255_Ad : Sum
  EMS_RollingCounter_id255_Convert : DataTypeConversion  OutDataTypeStr=uint32
  EMS_RollingCounter_id255_F : Gain
  EMS_RollingCounter_id255_L : simulink/Logic and Bit Operations/Bitwise Operator  logicop=AND  UseBitMask=on  BitMask=15  BitMaskRealWorld=Stored Integer
  EMS_RollingCounter_id255_O : Constant  Value=0  OutDataTypeStr=single
  EMS_RollingCounter_id255_S : ArithShift
  EMS_RollingCounter_id255_Sub : Subsystem
  EMS_RollingCounter_id255_sat : Saturate  UpperLimit=15  LowerLimit=0
  EMS_RollingCounter_id255cv : DataTypeConversion
  EMS_BrakePedalStatus_Out : Outport
  EMS_AccpedelError_Out : Outport  Port=2
  EMS_EngineSpeedError_Out : Outport  Port=3
  EMS_EngineSpeed_Out : Outport  Port=4
  EMS_AccPedal_Out : Outport  Port=5
  EMS_RollingCounter_id255_Out : Outport  Port=6
  EMS_CheckSum_255_Out : Outport  Port=7
  wires:
  EMS_BrakePedalStatus_F/1 -> EMS_BrakePedalStatus_Ad/1
  EMS_BrakePedalStatus_O/1 -> EMS_BrakePedalStatus_Ad/2
  EMS_BrakePedalStatus_Ad/1 -> EMS_BrakePedalStatus_sat/1
  EMS_BrakePedalStatus_sat/1 -> EMS_BrakePedalStatus_Out/1
  Demux/1 -> EMS_BrakePedalStatus_Sub/1(In1)
  EMS_BrakePedalStatus_Sub/1(Out1) -> EMS_BrakePedalStatus_Convert/1
  EMS_BrakePedalStatus_Convert/1 -> EMS_BrakePedalStatus_L/1
  EMS_BrakePedalStatus_L/1 -> EMS_BrakePedalStatus_S/1
  EMS_BrakePedalStatus_S/1 -> EMS_BrakePedalStatuscv/1
  EMS_BrakePedalStatuscv/1 -> EMS_BrakePedalStatus_F/1
  EMS_AccpedelError_F/1 -> EMS_AccpedelError_Ad/1
  EMS_AccpedelError_O/1 -> EMS_AccpedelError_Ad/2
  EMS_AccpedelError_Ad/1 -> EMS_AccpedelError_sat/1
  EMS_AccpedelError_sat/1 -> EMS_AccpedelError_Out/1
  Demux/2 -> EMS_AccpedelError_Sub/1(In1), EMS_EngineSpeedError_Sub/1(In1)
  EMS_AccpedelError_Sub/1(Out1) -> EMS_AccpedelError_Convert/1
  EMS_AccpedelError_Convert/1 -> EMS_AccpedelError_L/1
  EMS_AccpedelError_L/1 -> EMS_AccpedelError_S/1
  EMS_AccpedelError_S/1 -> EMS_AccpedelErrorcv/1
  EMS_AccpedelErrorcv/1 -> EMS_AccpedelError_F/1
  EMS_EngineSpeedError_F/1 -> EMS_EngineSpeedError_Ad/1
  EMS_EngineSpeedError_O/1 -> EMS_EngineSpeedError_Ad/2
  EMS_EngineSpeedError_Ad/1 -> EMS_EngineSpeedError_sat/1
  EMS_EngineSpeedError_sat/1 -> EMS_EngineSpeedError_Out/1
  EMS_EngineSpeedError_Sub/1(Out1) -> EMS_EngineSpeedError_Convert/1
  EMS_EngineSpeedError_Convert/1 -> EMS_EngineSpeedError_L/1
  EMS_EngineSpeedError_L/1 -> EMS_EngineSpeedError_S/1
  EMS_EngineSpeedError_S/1 -> EMS_EngineSpeedErrorcv/1
  EMS_EngineSpeedErrorcv/1 -> EMS_EngineSpeedError_F/1
  EMS_EngineSpeed_F/1 -> EMS_EngineSpeed_Ad/1
  EMS_EngineSpeed_O/1 -> EMS_EngineSpeed_Ad/2
  EMS_EngineSpeed_Ad/1 -> EMS_EngineSpeed_sat/1
  EMS_EngineSpeed_sat/1 -> EMS_EngineSpeed_Out/1
  Demux/3 -> EMS_EngineSpeedinput3_P/1
  EMS_EngineSpeedinput3_C/1 -> EMS_EngineSpeedinput3_P/2
  EMS_EngineSpeedinput3_P/1 -> EMS_EngineSpeedinput3_Ad/1
  Demux/4 -> EMS_EngineSpeedinput3_Ad/2
  EMS_EngineSpeedinput3_Ad/1 -> EMS_EngineSpeed_Sub/1(In1)
  EMS_EngineSpeed_Sub/1(Out1) -> EMS_EngineSpeed_Convert/1
  EMS_EngineSpeed_Convert/1 -> EMS_EngineSpeed_L/1
  EMS_EngineSpeed_L/1 -> EMS_EngineSpeed_S/1
  EMS_EngineSpeed_S/1 -> EMS_EngineSpeedcv/1
  EMS_EngineSpeedcv/1 -> EMS_EngineSpeed_F/1
  EMS_AccPedal_F/1 -> EMS_AccPedal_Ad/1
  EMS_AccPedal_O/1 -> EMS_AccPedal_Ad/2
  EMS_AccPedal_Ad/1 -> EMS_AccPedal_sat/1
  EMS_AccPedal_sat/1 -> EMS_AccPedal_Out/1
  Demux/6 -> EMS_AccPedal_Sub/1(In1)
  EMS_AccPedal_Sub/1(Out1) -> EMS_AccPedal_Convert/1
  EMS_AccPedal_Convert/1 -> EMS_AccPedal_L/1
  EMS_AccPedal_L/1 -> EMS_AccPedal_S/1
  EMS_AccPedal_S/1 -> EMS_AccPedalcv/1
  EMS_AccPedalcv/1 -> EMS_AccPedal_F/1
  EMS_RollingCounter_id255_F/1 -> EMS_RollingCounter_id255_Ad/1
  EMS_RollingCounter_id255_O/1 -> EMS_RollingCounter_id255_Ad/2
  EMS_RollingCounter_id255_Ad/1 -> EMS_RollingCounter_id255_sat/1
  EMS_RollingCounter_id255_sat/1 -> EMS_RollingCounter_id255_Out/1
  Demux/8 -> EMS_RollingCounter_id255_Sub/1(In1), EMS_CheckSum_255_Sub/1(In1)
  EMS_RollingCounter_id255_Sub/1(Out1) -> EMS_RollingCounter_id255_Convert/1
  EMS_RollingCounter_id255_Convert/1 -> EMS_RollingCounter_id255_L/1
  EMS_RollingCounter_id255_L/1 -> EMS_RollingCounter_id255_S/1
  EMS_RollingCounter_id255_S/1 -> EMS_RollingCounter_id255cv/1
  EMS_RollingCounter_id255cv/1 -> EMS_RollingCounter_id255_F/1
  EMS_CheckSum_255_F/1 -> EMS_CheckSum_255_Ad/1
  EMS_CheckSum_255_O/1 -> EMS_CheckSum_255_Ad/2
  EMS_CheckSum_255_Ad/1 -> EMS_CheckSum_255_sat/1
  EMS_CheckSum_255_sat/1 -> EMS_CheckSum_255_Out/1
  EMS_CheckSum_255_Sub/1(Out1) -> EMS_CheckSum_255_Convert/1
  EMS_CheckSum_255_Convert/1 -> EMS_CheckSum_255_L/1
  EMS_CheckSum_255_L/1 -> EMS_CheckSum_255_S/1
  EMS_CheckSum_255_S/1 -> EMS_CheckSum_255cv/1
  EMS_CheckSum_255cv/1 -> EMS_CheckSum_255_F/1
  input/1 -> Demux/1
